simulink library "test_library"  (Simulink 7.9)
settings: Solver=ode45  StartTime=0.0  StopTime=10.0  RelTol=1e-3
undefined symbols (not defined in the file): cputime, objectSelected, tUS_RHS
libraries: test_library x10, simulink x6
settings Model: Creator=falter  LastModifiedBy=falter

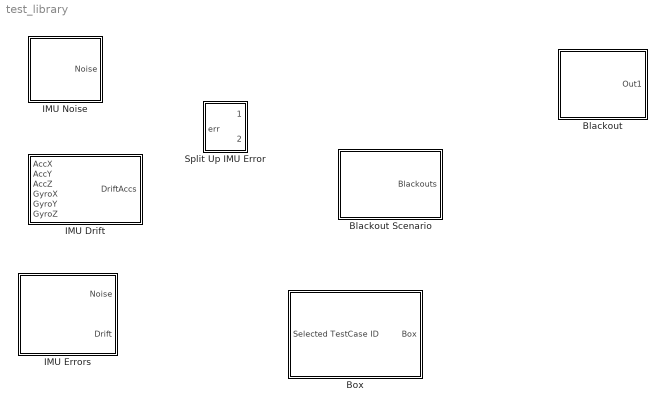
== system test_library ==
  Blackout : Subsystem  mask{t=tUS_RHS}
      mask prompts: t "Time of Blackout [seconds]"
      mask help:
      | Block to schedule sensor system blackout events.
      | The blackout occures after the number of seconds, specified as "Time of Blackout".
      | If -1 is set as time, there will not be a blackout event at all.
      mask Display:
      | fprintf('Time\nTiggered\nBlackout');
      | 
      | port_label('output', 1, 'bo');
  Blackout Scenario : Subsystem  mask{tAHRS=-1, tPMD=60, tUS_GND=-1, tUS_FRONT=-1, tUS_LHS=96, tUS_RHS=-1, tUS_CEIL=-1, tUS_REAR=-1}
      mask prompts: tAHRS "Blackout Time AHRS"; tPMD "Blackout Time PMD"; tUS_GND "Blackout Time Ultra Sonic Ground"; tUS_FRONT "Blackout Time Ultra Sonic Front"; tUS_LHS "Blackout Time Ultra Sonic LHS"; tUS_RHS "Blackout Time Ultra Sonic RHS"; tUS_CEIL "Blackout Time Ultra Sonic Ceiling"; tUS_REAR "Blackout Time Ultra Sonic Rear"
      mask help:
      | Specifiy simulation time in seconds, after which a blackout of the respective system shall occure.
      | Or '-1', if the System shall not fail.
      mask Display:
      | fprintf('Blackout\nScenario');
      | 
      | port_label('output',1,'Bo');
  Box : Subsystem  mask{t=1, p=[0, 0, 0], d=[1, 2, 3], tc_ids=[1 2]}
      mask prompts: t "Appearance Time"; p "Box Position"; d "Box Dimensions"; tc_ids "Belongs to Test Cases (Set of Numbers)"
      mask help:
      | Creates a Box with the given dimensinos at the given position after the given number of seconds.
      | By giving one or more scenario ids, the Box will be triggered for the corresponding obstacle scenarios.
      |
      | (This block also takes care about the visualization within the 3D simulation.)
      mask Display:
      | str = '';
      | 
      | for i = tc_ids,
      |     str = [str sprintf(' %d', i)];
      | end;
      | 
      | fprintf('TimedStaticBox\n\n(App.: %gs)\n\nTest Cases: %s', t, str);
      | 
      | port_label ('output', 1, 'B-Rep');
      | port_label ('input', 1, 'S. ID');
  IMU Drift : Subsystem
      mask Display:
      | fprintf('IMU\nDrift\nAccumu-\nlator');
      | 
      | port_label('output', 1, 'err');
      | 
      | port_label('input', 1, 'AccX');
      | port_label('input', 2, 'AccY');
      | port_label('input', 3, 'AccZ');
      | port_label('input', 4, 'GyroX');
      | port_label('input', 5, 'GyroY');
      | port_label('input', 6, 'GyroZ');
  IMU Errors : Subsystem  mask{tAHRS=-1, tLaser=-1, tPMD=-1, tUS_GND=-1, tUS_FRONT=-1, tUS_LHS=-1, tUS_RHS=-1, tUS_CEIL=-1, tUS_REAR=-1, nAccX=0, nAccY=0, nAccZ=0, dAccX=0, dAccY=0, dAccZ=0, nGyroX=0, nGyroY=0, nGyroZ=0, dGyroX=0, dGyroY=0, dGyroZ=0}
      mask prompts: tAHRS "AHRS Blackout Time"; tLaser "Laser Blackout Time"; tPMD "PMD Blackout Time"; tUS_GND "US GND Blackout Time"; tUS_FRONT "US FRONT Blackout Time"; tUS_LHS "US LHS Blackout Time"; tUS_RHS "US RHS Blackout Time"; tUS_CEIL "US CEILING Blackout Time"; tUS_REAR "US REAR Blackout Time"; nAccX "Max ACC X Noise"; nAccY "Max ACC Y Noise"; nAccZ "Max ACC Z Noise"; dAccX "Max ACC X Drift"; dAccY "Max ACC Y Drift"; dAccZ "Max ACC Z Drift"; nGyroX "Max Gyro X Noise"; nGyroY "Max Gyro Y Noise"; nGyroZ "MaxGyro Z Noise"; dGyroX "Max Gyro X Drift"; dGyroY "Max Gyro Y Drift"; dGyroZ "Max Gyro Z Drift"
      mask help:
      | Enter the Test Case parameters here.
      |
      | Specify the maximum absolute error for each of the IMU data components.
      mask Display:
      | fprintf('Sensor\nErrors');
      | 
      | port_label('output', 1, 'Noise');
      | port_label('output', 2, 'Drifts');
  IMU Noise : Subsystem  mask{accX=0, accY=0.025, accZ=0, gX=0, gY=0, gZ=0, sTime=0.01}
      mask prompts: accX "Max Noise Acc X"; accY "Max Noise Acc Y"; accZ "Max Noise Acc Z"; gX "Max Noise Gyro X"; gY "Max Noise Gyro Y"; gZ "Max Noise Gyro Z"; sTime "Sample Time"
      mask help: Specify maximum absolute error values for the IMU noise generation.
      mask Display:
      | fprintf('IMU\nNoise');
      | 
      | port_label('output', 1, 'err');
  Split Up IMU Error : Subsystem

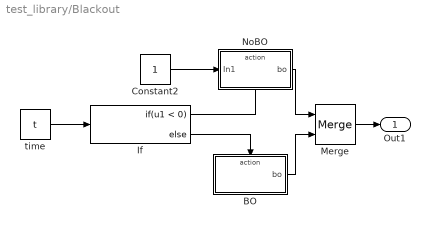
== system test_library/Blackout ==
  BO : Subsystem  TreatAsAtomicUnit=on
  Constant2 : Constant  VectorParams1D=off
  If : If  IfExpression=u1 < 0
  Merge : Merge
  NoBO : Subsystem  TreatAsAtomicUnit=on
  time : Constant  Value=t  VectorParams1D=off
  Out1 : Outport
  wires:
  Constant2/1 -> NoBO/1(In1)
  time/1 -> If/1
  Merge/1 -> Out1/1
  If/1 -> NoBO/Action
  If/2 -> BO/Action
  NoBO/1(bo) -> Merge/1
  BO/1(bo) -> Merge/2

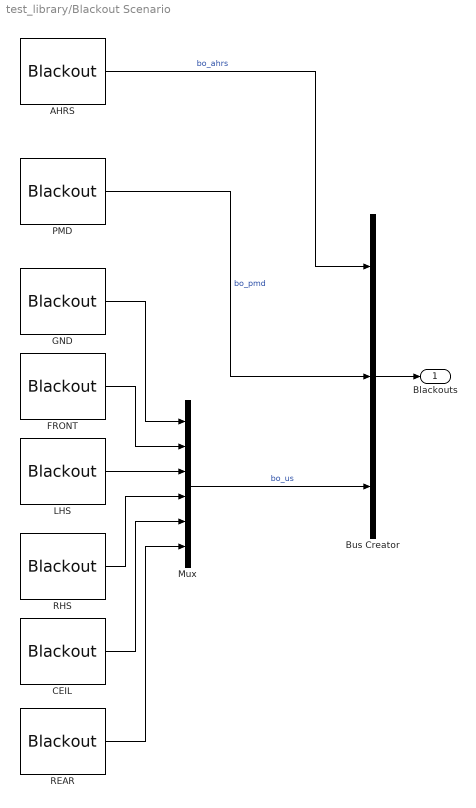
== system test_library/Blackout Scenario ==
  AHRS : test_library/Blackout  t=tAHRS
  Bus Creator : BusCreator  Inputs=3
  CEIL : test_library/Blackout  t=tUS_CEIL
  FRONT : test_library/Blackout  t=tUS_FRONT
  GND : test_library/Blackout  t=tUS_GND
  LHS : test_library/Blackout  t=tUS_LHS
  Mux : Mux  Inputs=6
  PMD : test_library/Blackout  t=tPMD
  REAR : test_library/Blackout  t=tUS_REAR
  RHS : test_library/Blackout  t=tUS_RHS
  Blackouts : Outport
  wires:
  Bus Creator/1 -> Blackouts/1
  AHRS/1 -> Bus Creator/1  "bo_ahrs"
  GND/1 -> Mux/1
  FRONT/1 -> Mux/2
  LHS/1 -> Mux/3
  RHS/1 -> Mux/4
  CEIL/1 -> Mux/5
  REAR/1 -> Mux/6
  PMD/1 -> Bus Creator/2  "bo_pmd"
  Mux/1 -> Bus Creator/3  "bo_us"

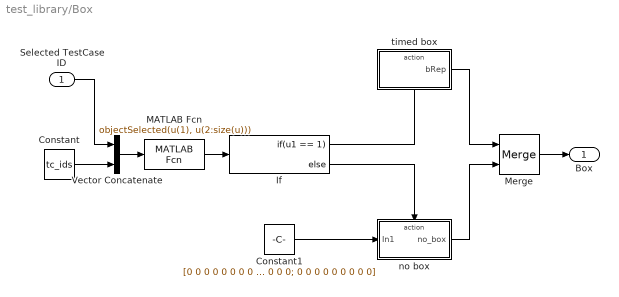
== system test_library/Box ==
  Selected TestCase ID : Inport
  Constant : Constant  Value=tc_ids
  Constant1 : Constant  Value=[0 0 0 0 0 0 0 0 0; 0 0 0 0 0 0 0 0 0; 0 0 0 0 0 0 0 0 0;0 0 0 0 0 0 0 0 0; 0 0 0 0 0 0 0 0 0; 0 0 0 0 0 0 0 0 0]
  If : If  IfExpression=u1 == 1
  MATLAB Fcn : MATLABFcn  MATLABFcn=objectSelected(u(1), u(2:size(u)))
  Merge : Merge  InitialOutput=[0 0 0 0 0 0 0 0 0; 0 0 0 0 0 0 0 0 0; 0 0 0 0 0 0 0 0 0;0 0 0 0 0 0 0 0 0; 0 0 0 0 0 0 0 0 0; 0 0 0 0 0 0 0 0 0]
  Vector Concatenate : Concatenate
  no box : Subsystem  TreatAsAtomicUnit=on
  timed box : Subsystem  TreatAsAtomicUnit=on
  Box : Outport
  wires:
  MATLAB Fcn/1 -> If/1
  Vector Concatenate/1 -> MATLAB Fcn/1
  Constant/1 -> Vector Concatenate/2
  Selected TestCase ID/1 -> Vector Concatenate/1
  If/1 -> timed box/Action
  If/2 -> no box/Action
  timed box/1(bRep) -> Merge/1
  no box/1(no_box) -> Merge/2
  Merge/1 -> Box/1
  Constant1/1 -> no box/1(In1)

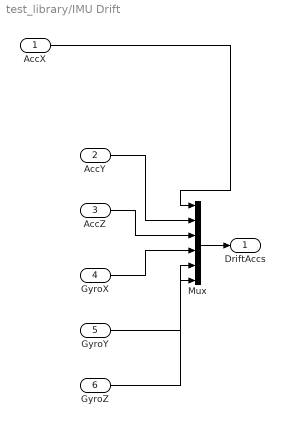
== system test_library/IMU Drift ==
  AccX : Inport
  AccY : Inport  Port=2
  AccZ : Inport  Port=3
  GyroX : Inport  Port=4
  GyroY : Inport  Port=5
  GyroZ : Inport  Port=6
  Mux : Mux  Inputs=6
  DriftAccs : Outport
  wires:
  GyroZ/1 -> Mux/6
  GyroY/1 -> Mux/5
  GyroX/1 -> Mux/4
  AccZ/1 -> Mux/3
  AccY/1 -> Mux/2
  AccX/1 -> Mux/1
  Mux/1 -> DriftAccs/1

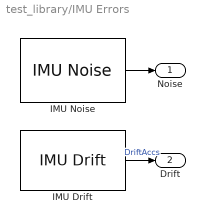
== system test_library/IMU Errors ==
  IMU Drift : test_library/IMU Drift  SystemSampleTime=-1
  IMU Noise : test_library/IMU Noise  SystemSampleTime=-1  accX=nAccX  accY=nAccY  accZ=nAccZ  gX=nGyroX  gY=nGyroY  gZ=nGyroZ
  Noise : Outport
  Drift : Outport  Port=2
  wires:
  IMU Noise/1 -> Noise/1
  IMU Drift/1 -> Drift/1  "DriftAccs"

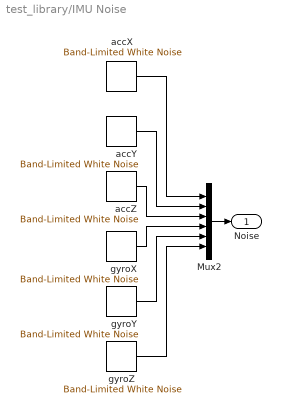
== system test_library/IMU Noise ==
  Mux2 : Mux  Inputs=6
  accX : simulink/Sources/Band-Limited White Noise  Cov=[accX]  Ts=sTime  seed=[round(cputime*1000)]
  accY : simulink/Sources/Band-Limited White Noise  Cov=[accY]  Ts=sTime  seed=[round(cputime*1000)]
  accZ : simulink/Sources/Band-Limited White Noise  Cov=[accZ]  Ts=sTime  seed=[round(cputime*1000)]
  gyroX : simulink/Sources/Band-Limited White Noise  Cov=[gX]  Ts=sTime  seed=[round(cputime*1000)]
  gyroY : simulink/Sources/Band-Limited White Noise  Cov=[gY]  Ts=sTime  seed=[round(cputime*1000)]
  gyroZ : simulink/Sources/Band-Limited White Noise  Cov=[gZ]  Ts=sTime  seed=[round(cputime*1000)]
  Noise : Outport
  wires:
  gyroX/1 -> Mux2/4
  gyroY/1 -> Mux2/5
  gyroZ/1 -> Mux2/6
  accZ/1 -> Mux2/3
  accY/1 -> Mux2/2
  accX/1 -> Mux2/1
  Mux2/1 -> Noise/1

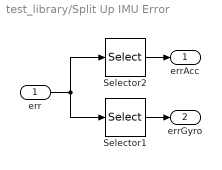
== system test_library/Split Up IMU Error ==
  err : Inport
  Selector1 : Selector  InputPortWidth=6  IndexOptions=Index vector (dialog)  Indices=[4 5 6]  OutputSizes=1
  Selector2 : Selector  InputPortWidth=6  IndexOptions=Index vector (dialog)  Indices=[1 2 3]  OutputSizes=1
  errAcc : Outport
  errGyro : Outport  Port=2
  wires:
  err/1 -> Selector1/1, Selector2/1
  Selector2/1 -> errAcc/1
  Selector1/1 -> errGyro/1

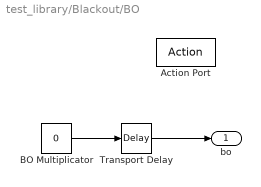
== system test_library/Blackout/BO ==
  Action Port : ActionPort
  BO Multiplicator : Constant  Value=0  VectorParams1D=off
  Transport Delay : TransportDelay  DelayTime=abs(t)  InitialOutput=1  BufferSize=16384
  bo : Outport
  wires:
  BO Multiplicator/1 -> Transport Delay/1
  Transport Delay/1 -> bo/1

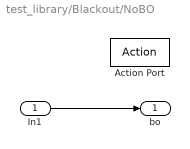
== system test_library/Blackout/NoBO ==
  In1 : Inport
  Action Port : ActionPort
  bo : Outport
  wires:
  In1/1 -> bo/1

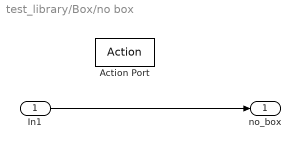
== system test_library/Box/no box ==
  In1 : Inport
  Action Port : ActionPort
  no_box : Outport
  wires:
  In1/1 -> no_box/1

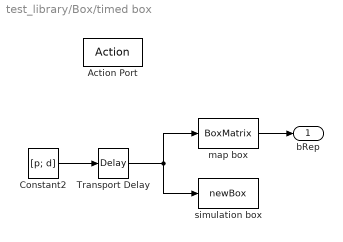
== system test_library/Box/timed box ==
  Action Port : ActionPort
  Constant2 : Constant  Value=[p; d]  VectorParams1D=off
  Transport Delay : TransportDelay  DelayTime=t  BufferSize=18432
  map box : MATLABFcn  MATLABFcn=BoxMatrix  OutputDimensions=[6, 9]  Output1D=off
  simulation box : MATLABFcn  MATLABFcn=newBox  OutputDimensions=0  Output1D=off
  bRep : Outport
  wires:
  map box/1 -> bRep/1
  Transport Delay/1 -> simulation box/1, map box/1
  Constant2/1 -> Transport Delay/1
